simulink model "FSFB_MO_DoublePendulum"  (R2023b)
settings: Solver=VariableStepAuto  StartTime=0.0  StopTime=10.0  RelTol=1e-3
values from neighbouring files (symbols this model uses):
  A = [0 1 0 0; 9.8 0 -9.8 0; 0 0 0 1; -9.8 0 2.94 0]    [FSFB_FO_MIMO_doublePendulum.m]    (also in FSFB_MIMO_doublePendulum.m; FSFB_MO_MIMO_doublePendulum.m)
  B = [0 0; 1 -2; 0 0; -2 5]    [FSFB_FO_MIMO_doublePendulum.m]    (also in FSFB_MIMO_doublePendulum.m; FSFB_MO_MIMO_doublePendulum.m)
  C = [1 0 0 0; 0 0 1 0]    [FSFB_FO_MIMO_doublePendulum.m]    (also in FSFB_MIMO_doublePendulum.m; FSFB_MO_MIMO_doublePendulum.m)
  Inversa_MA = Ma^-1    [FSFB_MO_MIMO_doublePendulum.m]
  K_moore = W_moore/V_moore    [FSFB_FO_MIMO_doublePendulum.m]    (also in FSFB_MIMO_doublePendulum.m; FSFB_MO_MIMO_doublePendulum.m)
  MatrizPI = diag(polos_desejados_observador_rapido)    [FSFB_MO_MIMO_doublePendulum.m]
  Q_moore = qr    [FSFB_FO_MIMO_doublePendulum.m]    (also in FSFB_MO_MIMO_doublePendulum.m = -q)
  T = [[0 1 1 -1]' [1 1 -1 0]']    [FSFB_FO_MIMO_doublePendulum.m]    (also in FSFB_MO_MIMO_doublePendulum.m = -[[0 1]; [1 1]])
  x0 = [0 1 0 1]    [FSFB_FO_MIMO_doublePendulum.m]    (also in FSFB_MIMO_doublePendulum.m; FSFB_MO_MIMO_doublePendulum.m)
settings Model: Creator=frede  LastModifiedBy=frede

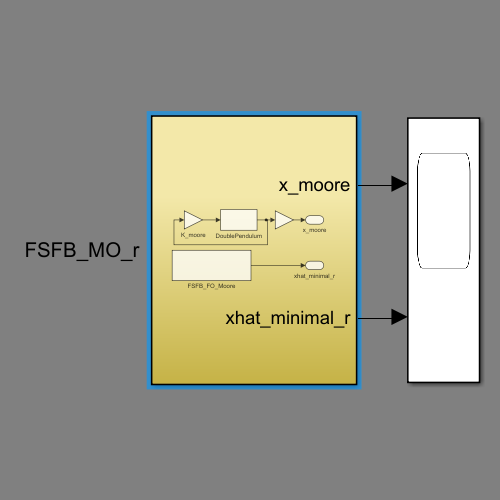
[thumbnail: Simulink's stored preview of the top-level diagram]
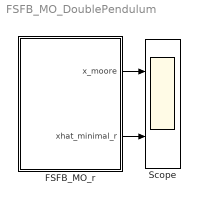
== system FSFB_MO_DoublePendulum ==
  FSFB_MO_r : Subsystem
  Scope : Scope  NumInputPorts=2
  wires:
  FSFB_MO_r/1(x_moore) -> Scope/1
  FSFB_MO_r/2(xhat_minimal_r) -> Scope/2

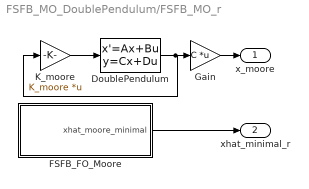
== system FSFB_MO_DoublePendulum/FSFB_MO_r ==
  DoublePendulum : StateSpace  A=A  B=B  C=eye(4)  D=zeros(4, 2)  InitialCondition=x0
  FSFB_FO_Moore : Subsystem
  Gain : Gain  Gain=C  Multiplication=Matrix(K*u)
  K_moore : Gain  Gain=K_moore  Multiplication=Matrix(K*u) (u vector)
  x_moore : Outport
  xhat_minimal_r : Outport  Port=2
  wires:
  K_moore/1 -> DoublePendulum/1
  DoublePendulum/1 -> K_moore/1, Gain/1
  FSFB_FO_Moore/1(xhat_moore_minimal) -> xhat_minimal_r/1
  Gain/1 -> x_moore/1

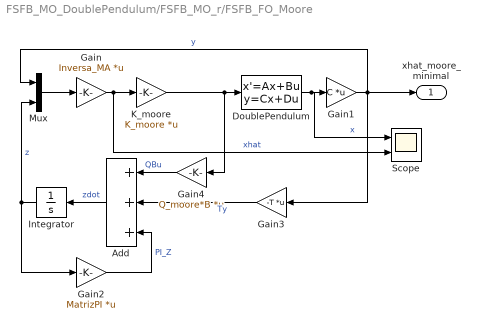
== system FSFB_MO_DoublePendulum/FSFB_MO_r/FSFB_FO_Moore ==
  Add : Sum  Inputs=+++
  "DoublePendulum  " : StateSpace  A=A  B=B  C=eye(4)  D=zeros(4, 2)  InitialCondition=x0
  Gain : Gain  Gain=Inversa_MA  Multiplication=Matrix(K*u) (u vector)
  Gain1 : Gain  Gain=C  Multiplication=Matrix(K*u) (u vector)
  Gain2 : Gain  Gain=MatrizPI  Multiplication=Matrix(K*u) (u vector)
  Gain3 : Gain  Gain=-T  Multiplication=Matrix(K*u) (u vector)
  Gain4 : Gain  Gain=Q_moore*B  Multiplication=Matrix(K*u) (u vector)
  Integrator : Integrator
  K_moore : Gain  Gain=K_moore  Multiplication=Matrix(K*u) (u vector)
  Mux : Mux  Inputs=2
  Scope : Scope  NumInputPorts=2
  xhat_moore_minimal : Outport
  wires:
  "DoublePendulum  "/1 -> Gain1/1, Scope/1  "x"
  K_moore/1 -> Gain4/1, "DoublePendulum  "/1
  Gain1/1 -> Mux/1, Gain3/1, xhat_moore_minimal/1  "y"
  Gain/1 -> Scope/2, K_moore/1  "xhat"
  Mux/1 -> Gain/1
  Integrator/1 -> Mux/2, Gain2/1  "z"
  Add/1 -> Integrator/1  "zdot"
  Gain2/1 -> Add/3  "PI_Z"
  Gain3/1 -> Add/2  "Ty"
  Gain4/1 -> Add/1  "QBu"
